simulink model "Single_track"  (Simulink 8.6)
settings: Solver=ode45  StartTime=0.0  StopTime=10.0  RelTol=1e-3
values from neighbouring files (symbols this model uses):
  a11 = (-1/v)*((Caf*Lf^2+Car*Lr^2)/Th)    (= -7.16694716187)    [Single_track_ini.m]
  a12 = -((Caf*Lf-Car*Lr)/Th)    (= 6.07923243578)    [Single_track_ini.m]
  a21 = (-1-((1/v^2)*((Caf*Lf-Car*Lr)/m)))    (= -0.90501934236)    [Single_track_ini.m]
  a22 = (-1/v)*((Caf+Car)/m)    (= -6.28626692456)    [Single_track_ini.m]
  b1 = 1/Th    (= 0.000309501702259)    [Single_track_ini.m]
  b2 = 0    [Single_track_ini.m]
libraries: simulink x1
settings Model: Creator=jasper.desmet  LastModifiedBy=MVdB
settings OptimizationCC: InitFltsAndDblsToZero=on
settings DebuggingCC: FcnCallInpInsideContextMsg=UseLocalSettings
settings GRTTargetCC: GeneratePreprocessorConditionals=Use local settings

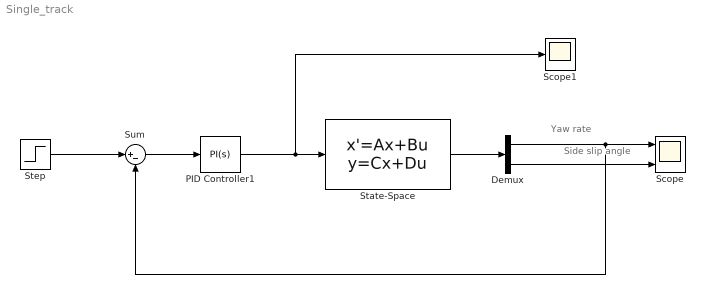
== system Single_track ==
  note: Yaw rate
  note: Side slip angle
  Demux : Demux  Outputs=2
  PID Controller1 : simulink/Continuous/PID Controller  Controller=PI  TimeDomain=Continuous-time  SampleTime=-1  IntegratorMethod=Forward Euler  FilterMethod=Forward Euler  Form=Parallel  UseFilter=on  ControllerParametersSource=internal  P=353.332221657154  I=144713.569417884  D=-291.19831355653  N=1036.52333286906  InitialConditionSource=internal  InitialConditionForIntegrator=0  InitialConditionForFilter=0  ExternalReset=none  LimitOutput=off  UpperSaturationLimit=inf  LowerSaturationLimit=-inf  LinearizeAsGain=on  AntiWindupMode=none  Kb=1  TrackingMode=off  Kt=1  PParamMin=[]  PParamMax=[]  IParamMin=[]  IParamMax=[]  DParamMin=[]  DParamMax=[]  NParamMin=[]  NParamMax=[]  KbParamMin=[]  KbParamMax=[]  KtParamMin=[]  KtParamMax=[]  POutMin=[]  POutMax=[]  IOutMin=[]  IOutMax=[]  DOutMin=[]  DOutMax=[]  NOutMin=[]  NOutMax=[]  KbOutMin=[]  KbOutMax=[]  KtOutMin=[]  KtOutMax=[]  IntegratorOutMin=[]  IntegratorOutMax=[]  FilterOutMin=[]  FilterOutMax=[]  SumOutMin=[]  SumOutMax=[]  SumI1OutMin=[]  SumI1OutMax=[]  SumI2OutMin=[]  SumI2OutMax=[]  SumI3OutMin=[]  SumI3OutMax=[]  SumDOutMin=[]  SumDOutMax=[]  SaturationOutMin=[]  SaturationOutMax=[]  IntegratorContinuousStateAttributes=''  IntegratorStateMustResolveToSignalObject=off  IntegratorRTWStateStorageClass=Auto  FilterContinuousStateAttributes=''  FilterStateMustResolveToSignalObject=off  FilterRTWStateStorageClass=Auto  DifferentiatorICPrevScaledInput=0  DifferentiatorOutMin=[]  DifferentiatorOutMax=[]
  Scope : Scope  NumInputPorts=2
  Scope1 : Scope
  State-Space : StateSpace  A=[a11 a12; a21 a22]  B=[b1; b2]  C=[1 0; 0 1]  D=[0; 0]  X0=0
  Step : Step  Time=3  SampleTime=0
  Sum : Sum  Inputs=|+-
  wires:
  State-Space/1 -> Demux/1
  Demux/1 -> Scope/1, Sum/2
  Demux/2 -> Scope/2
  Step/1 -> Sum/1
  PID Controller1/1 -> State-Space/1, Scope1/1
  Sum/1 -> PID Controller1/1
